simulink model "Ex2"  (R2019a)
settings: Solver=VariableStepAuto  StartTime=0.0  StopTime=10.0  RelTol=1e-3
values from neighbouring files (symbols this model uses):
  G = tf([1], [1 0.2683 5])    [Ex1.m]
undefined symbols (not defined in the file or in its folder): A, B, C, K
settings Model: Creator=sselvaraja2018  LastModifiedBy=sselvaraja2018

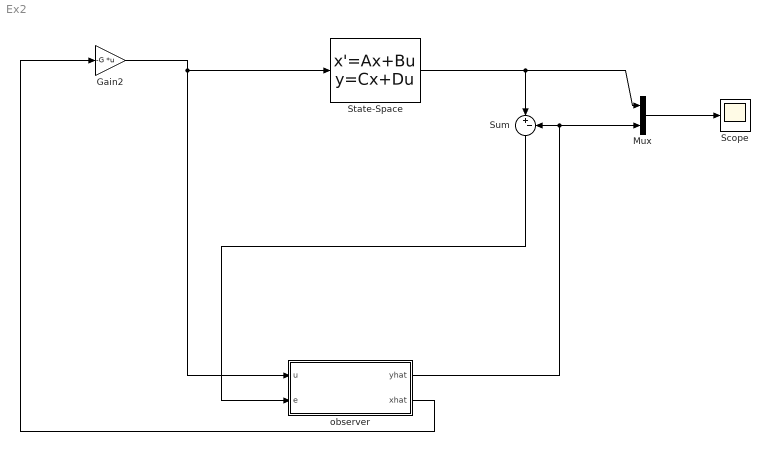
== system Ex2 ==
  " observer" : Subsystem
  Gain2 : Gain  Gain=-G  Multiplication=Matrix(K*u)
  Mux : Mux  Inputs=2
  Scope : Scope
  State-Space : StateSpace  A=[-0.01357 -32.2 -46.3 0; 0.00012 0 1.214 0; -0.0001212 0 -1.214 1; 0.00057 0 -0.1 -0.6696]  B=[-0.433;0.1394; -0.1394; -0.1577]  C=[0 0 0 1; 1 0 0 0]  D=[0; 0]  InitialCondition="[2 2 0  -1]"
  Sum : Sum  Inputs=|+-
  wires:
  State-Space/1 -> Sum/1, Mux/1
  Gain2/1 -> " observer"/1(u), State-Space/1
  Sum/1 -> " observer"/2(e)
  " observer"/1(yhat) -> Sum/2, Mux/2
  " observer"/2(xhat) -> Gain2/1
  Mux/1 -> Scope/1

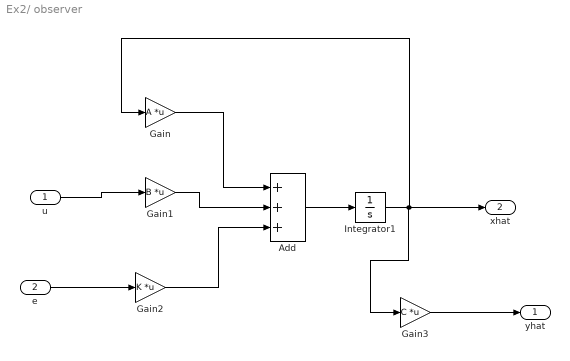
== system Ex2/ observer ==
  u : Inport
  e : Inport  Port=2
  Add : Sum  Inputs=+++
  Gain : Gain  Gain=A  Multiplication=Matrix(K*u)
  Gain1 : Gain  Gain=B  Multiplication=Matrix(K*u)
  Gain2 : Gain  Gain=K  Multiplication=Matrix(K*u)
  Gain3 : Gain  Gain=C  Multiplication=Matrix(K*u)
  Integrator1 : Integrator  InitialCondition=[2 2 0 -1]
  yhat : Outport
  xhat : Outport  Port=2
  wires:
  Gain1/1 -> Add/2
  Integrator1/1 -> xhat/1, Gain/1, Gain3/1
  u/1 -> Gain1/1
  Add/1 -> Integrator1/1
  Gain2/1 -> Add/3
  Gain/1 -> Add/1
  e/1 -> Gain2/1
  Gain3/1 -> yhat/1
